simulink model "ChiefMaster_TTC580"  (R2022b)
settings: Solver=FixedStepAuto  StartTime=0.0  StopTime=10  FixedStep=0.01  RelTol=1e-3
values from neighbouring files (symbols this model uses):
  BattBox1_No = single(1)    [Parameters.m]
  BattBox2_No = single(2)    [Parameters.m]
  BattBox3_No = single(3)    [Parameters.m]
  CurrentLB = single(-3)    [Parameters.m]
  CurrentReductionConstant_Lvl0 = single(0.03)    [Parameters.m]
  CurrentReductionConstant_Lvl1 = single(0.05)    [Parameters.m]
  CurrentReductionConstant_Lvl2 = single(0.07)    [Parameters.m]
  CurrentReductionConstant_Lvl3 = single(0.1)    [Parameters.m]
  CurrentUB = single(3)    [Parameters.m]
  DCHV_Minus_In_Delay_ms = single(500)    [Parameters.m]
  FL_sHVC_CellBalanceVoltage_mV = single(3500)    [Parameters.m]
  FL_sInrushCurrent_dividebyzero = single(0.00001)    [Parameters.m]
  FL_u8HMI_BuzzerTimer = uint8(3)    [Parameters.m]
  IP_boActValue = true    [Parameters.m]
  IP_boDeactValue = false    [Parameters.m]
  IP_boInitValue = false    [Parameters.m]
  IP_s_LB = 18000    [Parameters.m]
  IP_s_UB = 22000    [Parameters.m]
  IP_sBatt1_ChargeCurrentMax_Factor = single(0.1)    [Parameters.m]
  IP_sBatt1_ChargeCurrentMax_LB = single(0)    [Parameters.m]
  IP_sBatt1_ChargeCurrentMax_Offset = single(0)    [Parameters.m]
  IP_sBatt1_ChargeCurrentMax_UB = single(6553.5)    [Parameters.m]
  IP_sBatt1_Current_Factor = single(0.1)    [Parameters.m]
  IP_sBatt1_Current_LB = single(-3276.8)    [Parameters.m]
  IP_sBatt1_Current_Offset = single(0)    [Parameters.m]
  IP_sBatt1_Current_UB = single(3276.8)    [Parameters.m]
  IP_sBatt1_DisChargeCurrentMax_Factor = single(0.1)    [Parameters.m]
  IP_sBatt1_DisChargeCurrentMax_LB = single(0)    [Parameters.m]
  IP_sBatt1_DisChargeCurrentMax_Offset = single(0)    [Parameters.m]
  IP_sBatt1_DisChargeCurrentMax_UB = single(6553.5)    [Parameters.m]
  IP_sBatt1_InsulationResistance_Factor = single(5)    [Parameters.m]
  IP_sBatt1_InsulationResistance_LB = single(0)    [Parameters.m]
  IP_sBatt1_InsulationResistance_Offset = single(0)    [Parameters.m]
  IP_sBatt1_InsulationResistance_UB = single(0)    [Parameters.m]
  IP_sBatt1_LiBa_IntResist_mOhm = single(25)    [Parameters.m]
  IP_sBatt1_SOC_Factor = single(1)    [Parameters.m]
  IP_sBatt1_SOC_LB = single(0)    [Parameters.m]
  IP_sBatt1_SOC_Offset = single(0)    [Parameters.m]
  IP_sBatt1_SOC_UB = single(100)    [Parameters.m]
  IP_sBatt1_SOH_Factor = single(1)    [Parameters.m]
  IP_sBatt1_SOH_LB = single(0)    [Parameters.m]
  IP_sBatt1_SOH_Offset = single(0)    [Parameters.m]
  IP_sBatt1_SOH_UB = single(100)    [Parameters.m]
  IP_sBatt1_Ubatt_Factor = single(0.1)    [Parameters.m]
  IP_sBatt1_Ubatt_LB = single(0)    [Parameters.m]
  IP_sBatt1_Ubatt_Offset = single(0)    [Parameters.m]
  IP_sBatt1_Ubatt_UB = single(6553.5)    [Parameters.m]
  IP_sBatt1_UserRi_Factor = single(1)    [Parameters.m]
  IP_sBatt1_UserRi_LB = single(0)    [Parameters.m]
  IP_sBatt1_UserRi_Offset = single(0)    [Parameters.m]
  IP_sBatt1_UserRi_UB = single(255)    [Parameters.m]
  IP_sBatt1_VoltageAtSensor_Factor = single(0.02)    [Parameters.m]
  IP_sBatt1_VoltageAtSensor_LB = single(0)    [Parameters.m]
  IP_sBatt1_VoltageAtSensor_Offset = single(0)    [Parameters.m]
  IP_sBatt1_VoltageAtSensor_UB = single(1310.7)    [Parameters.m]
  IP_sBatt2_LiBa_IntResist_mOhm = single(25)    [Parameters.m]
  IP_sBatt3_LiBa_IntResist_mOhm = single(25)    [Parameters.m]
  IP_sEM_LB = 2000    [Parameters.m]
  IP_sEM_UB = 8000    [Parameters.m]
  IP_sFB_LB = 5000    [Parameters.m]
  IP_sFB_UB = 10000    [Parameters.m]
  IP_sHVIL_LB = 12000    [Parameters.m]
  IP_sHVIL_UB = 15000    [Parameters.m]
  IP_sLoad_Voltage_Factor = single(1)    [Parameters.m]
  IP_sLoad_Voltage_LB = single(0)    [Parameters.m]
  IP_sLoad_Voltage_Offset = single(0)    [Parameters.m]
  IP_sLoad_Voltage_UB = single(65535)    [Parameters.m]
  IP_u8HVIL_Delay_ms = uint8(100)    [Parameters.m]
  IP_u8HW_IN_delay_ms = uint8(100)    [Parameters.m]
  IT_sInsulationSafeValue_kOhm = single(650)    [Parameters.m]
  IT_u8IMD_DelayTime_s = uint8(20)    [Parameters.m]
  MainHV_Minus_In_Delay = single(5)    [Parameters.m]
  MainHV_StatusDelay = single(5)    [Parameters.m]
  NotAvailable_uint16 = single(65535)    [Parameters.m]
  NotAvailable_uint8 = uint8(255)    [Parameters.m]
  OP_boHVIL_Supply = boolean(1)    [Parameters.m]
  SafeCurrentToCloseHV_A = single(5)    [Parameters.m]
  SafeVoltageToCloseHV_V = single(0.5)    [Parameters.m]
  UnexpectedBattChargingFcn_Available = boolean(1)    [Parameters.m]
  Voltage_NA_UB = uint16(65535)    [Parameters.m]
  VoltageSensorAvailableBB1 = boolean(0)    [Parameters.m]
  VoltageSensorAvailableBB2 = boolean(0)    [Parameters.m]
  VoltageSensorAvailableBB3 = boolean(0)    [Parameters.m]
libraries: simulink x184, Library_DataProcessing_v1_1 x167, Library_DataProcessing_v1 x142, libCM x28
(part 4 of 19)

== system ChiefMaster_TTC580/ChiefMaster/Input Translation/HW Inputs ==
  IP_Databus : Inport
  Bus Creator : BusCreator  Inputs=15
  Bus Selector : BusSelector  OutputSignals=IP_HW_Input_DataBus.IP_boHW_KL15,IP_HW_Input_DataBus.IP_boHW_HVIL_BDU,IP_HW_Input_DataBus.IP_boHW_HVIL_Components,IP_HW_Input_DataBus.IP_boHW_HVIL_Battery,IP_HW_Input_DataBus.IP_boHW_HVIL_Overrule,IP_HW_Input_DataBus.IP_boHW_MainHV_Plus_FB,IP_HW_Input_DataBus.IP_boHW_MainHV_Minus_FB,IP_HW_Input_DataBus.IP_boHW_EmergencyButton_NC,IP_HW_Input_DataBus.IP_boHW_EmergencyButton_NO,IP_HW_Input_DataBus.IP_boHW_ResetButton_LED_NO,IP_HW_Input_DataBus.IP_boHW_Proximity_BB1,IP_HW_Input_DataBus.IP_boHW_Proximity_BB2,IP_HW_Input_DataBus.IP_boHW_Proximity_BB3,IP_HW_Input_DataBus.IP_boHW_DCHV_Plus_FB,IP_HW_Input_DataBus.IP_boHW_DCHV_Minus_FB
  Signal Copy{,1..14} (15 alike) : SignalConversion  OverrideOpt=off
  IT_HW_Input_Databus : Outport
  wires:
  Signal Copy/1 -> Bus Creator/1  "IT_boHW_KL15"
  Signal Copy11/1 -> Bus Creator/13  "IT_boHW_Proximity_BB3"
  Bus Selector/8 -> Signal Copy6/1  "<IP_boHW_EmergencyButton_NC>"
  Bus Selector/4 -> Signal Copy3/1  "<IP_boHW_HVIL_Battery>"
  Signal Copy3/1 -> Bus Creator/4  "IT_boHW_HVIL_Battery"
  Bus Selector/10 -> Signal Copy8/1  "<IP_boHW_ResetButton_LED_NO>"
  Signal Copy9/1 -> Bus Creator/11  "IT_boHW_Proximity_BB1"
  Signal Copy1/1 -> Bus Creator/2  "IT_boHW_HVIL_BDU"
  Signal Copy4/1 -> Bus Creator/6  "IT_boHW_MainHV_Plus_FB"
  Signal Copy2/1 -> Bus Creator/3  "IT_boHW_HVIL_Components"
  Bus Selector/15 -> Signal Copy13/1  "<IP_boHW_DCHV_Minus_FB>"
  Signal Copy6/1 -> Bus Creator/8  "IT_sHW_EmergencyButton_NC"
  Bus Selector/6 -> Signal Copy4/1  "<IP_boHW_MainHV_Plus_FB>"
  Bus Selector/7 -> Signal Copy5/1  "<IP_boHW_MainHV_Minus_FB>"
  Bus Selector/12 -> Signal Copy10/1  "<IP_boHW_Proximity_BB2>"
  Bus Selector/3 -> Signal Copy2/1  "<IP_boHW_HVIL_Components>"
  Signal Copy12/1 -> Bus Creator/14  "IT_boHW_DCHV_Plus_FB"
  Signal Copy5/1 -> Bus Creator/7  "IT_boHW_MainHV_Minus_FB"
  Signal Copy13/1 -> Bus Creator/15  "IT_boHW_DCHV_Minus_FB"
  Bus Selector/9 -> Signal Copy7/1  "<IP_boHW_EmergencyButton_NO>"
  Bus Selector/11 -> Signal Copy9/1  "<IP_boHW_Proximity_BB1>"
  Bus Selector/14 -> Signal Copy12/1  "<IP_boHW_DCHV_Plus_FB>"
  Bus Selector/13 -> Signal Copy11/1  "<IP_boHW_Proximity_BB3>"
  Signal Copy10/1 -> Bus Creator/12  "IT_boHW_Proximity_BB2"
  Bus Selector/1 -> Signal Copy/1  "<IP_boHW_KL15>"
  Signal Copy7/1 -> Bus Creator/9  "IT_boHW_EmergencyButton_NO"
  Bus Selector/2 -> Signal Copy1/1  "<IP_boHW_HVIL_BDU>"
  Signal Copy8/1 -> Bus Creator/10  "IT_boHW_ResetButton_LED_NO"
  IP_Databus/1 -> Bus Selector/1
  Bus Creator/1 -> IT_HW_Input_Databus/1  "IT_HW_Input_Databus"
  Bus Selector/5 -> Signal Copy14/1  "<IP_boHW_HVIL_Overrule>"
  Signal Copy14/1 -> Bus Creator/5  "IT_boHW_HVIL_Overrule"

== system ChiefMaster_TTC580/ChiefMaster/Input Translation/UDC ==
  IP_Databus : Inport
  Bus Creator : BusCreator  Inputs=7
  Bus Selector : BusSelector  OutputSignals=UDC_Databus.IP_UDC_Status_Databus.IP_boSafeToShutdown,UDC_Databus.IP_UDC_Status_Databus.IP_boKL15_D,UDC_Databus.IP_UDC_Status_Databus.IP_boKL15_C,UDC_Databus.IP_UDC_Status_Databus.IP_boEVDisconnectingDevice,UDC_Databus.IP_UDC_Status_Databus.IP_boEV_IsolationMeasurementRequest,UDC_Databus.IP_UDC_Status_Databus.IP_boChargeStop_Button,UDC_Databus.IP_sLoadVoltage_Databus
  Bus Selector1 : BusSelector  OutputSignals=sData
  Signal Copy{,1..6} (7 alike) : SignalConversion  OverrideOpt=off
  IT_UDC_Databus : Outport
  wires:
  Bus Selector/1 -> Signal Copy/1  "<IP_boSafeToShutdown>"
  Signal Copy/1 -> Bus Creator/1  "IT_boUDC_SafeToShutdown"
  Bus Selector/3 -> Signal Copy2/1  "<IP_boKL15_C>"
  Signal Copy1/1 -> Bus Creator/2  "IT_boUDC_KL15_D"
  Bus Selector/2 -> Signal Copy1/1  "<IP_boKL15_D>"
  IP_Databus/1 -> Bus Selector/1
  Bus Selector1/1 -> Signal Copy3/1  "<sData>"
  Bus Selector/7 -> Bus Selector1/1  "<IP_sLoadVoltage_Databus>"
  Signal Copy2/1 -> Bus Creator/3  "IT_boUDC_KL15_C"
  Signal Copy3/1 -> Bus Creator/7  "IT_sUDC_LoadVoltage_V"
  Bus Creator/1 -> IT_UDC_Databus/1  "IT_UDC_Databus"
  Bus Selector/4 -> Signal Copy4/1  "<IP_boEVDisconnectingDevice>"
  Signal Copy4/1 -> Bus Creator/4  "IT_boUDC_EVDisconnectingDevice"
  Bus Selector/5 -> Signal Copy5/1  "<IP_boEV_IsolationMeasurementRequest>"
  Signal Copy5/1 -> Bus Creator/5  "IT_boUDC_EV_IsolationMeasurementRequest"
  Bus Selector/6 -> Signal Copy6/1  "<IP_boChargeStop_Button>"
  Signal Copy6/1 -> Bus Creator/6  "IT_boChargeStop_Button"

== system ChiefMaster_TTC580/ChiefMaster/Output Processing/CM_OBD ==
  OT_Databus : Inport
  CM_BDU_Msg5_6 : Subsystem
  CM_Battery1_Msg7 : Subsystem
  CM_Battery1_Msg8 : Subsystem
  CM_Battery1_Msg9 : Subsystem
  CM_Battery2_Msg10 : Subsystem
  CM_Battery2_Msg11 : Subsystem
  CM_Battery2_Msg12 : Subsystem
  CM_Battery3_Msg13 : Subsystem
  CM_Battery3_Msg14 : Subsystem
  CM_Battery3_Msg15 : Subsystem
  CM_IP_Msg1 : Subsystem
  CM_OP_Msg2 : Subsystem
  CM_SystemStatus1_Msg3 : Subsystem
  CM_SystemStatus2_Msg4 : Subsystem
  OP_ChiefMaster_IP_Msg1 : Outport
  OP_ChiefMaster_OP_Msg2 : Outport  Port=2
  OP_ChiefMaster_SS1_Msg3 : Outport  Port=3
  OP_ChiefMaster_SS2_Msg4 : Outport  Port=4
  OP_ChiefMaster_Calc_Msg5 : Outport  Port=5
  OP_ChiefMaster_BDU_Msg6 : Outport  Port=6
  OP_ChiefMaster_Battery1_Msg7 : Outport  Port=7
  OP_ChiefMaster_Battery1_Msg8 : Outport  Port=8
  OP_ChiefMaster_Battery1_Msg9 : Outport  Port=9
  OP_ChiefMaster_Battery2_Msg10 : Outport  Port=10
  OP_ChiefMaster_Battery2_Msg11 : Outport  Port=11
  OP_ChiefMaster_Battery2_Msg12 : Outport  Port=12
  OP_ChiefMaster_Battery3_Msg13 : Outport  Port=13
  OP_ChiefMaster_Battery3_Msg14 : Outport  Port=14
  OP_ChiefMaster_Battery3_Msg15 : Outport  Port=15
  wires:
  CM_SystemStatus1_Msg3/1(OP_ChiefMaster_SS_Msg3) -> OP_ChiefMaster_SS1_Msg3/1
  CM_SystemStatus2_Msg4/1(OP_ChiefMaster_SS2_Msg4) -> OP_ChiefMaster_SS2_Msg4/1
  CM_IP_Msg1/1(OP_ChiefMaster_IP_Msg1) -> OP_ChiefMaster_IP_Msg1/1
  CM_OP_Msg2/1(OP_ChiefMaster_OP_Msg2) -> OP_ChiefMaster_OP_Msg2/1
  CM_BDU_Msg5_6/1("Chief_Master_Calc_Msg5 ") -> OP_ChiefMaster_Calc_Msg5/1
  CM_BDU_Msg5_6/2(Chief_Master_BDU_Msg6) -> OP_ChiefMaster_BDU_Msg6/1
  CM_Battery1_Msg7/1(OP_ChiefMaster_Battery1_Msg7) -> OP_ChiefMaster_Battery1_Msg7/1
  CM_Battery1_Msg8/1(OP_ChiefMaster_Battery1_Msg8) -> OP_ChiefMaster_Battery1_Msg8/1
  CM_Battery2_Msg11/1(OP_ChiefMaster_Battery2_Msg10) -> OP_ChiefMaster_Battery2_Msg11/1
  CM_Battery2_Msg10/1(OP_ChiefMaster_Battery2_Msg9) -> OP_ChiefMaster_Battery2_Msg10/1
  OT_Databus/1 -> CM_IP_Msg1/1(OT_Databus), CM_OP_Msg2/1(OT_Databus), CM_SystemStatus1_Msg3/1(OT_Databus), CM_SystemStatus2_Msg4/1(OT_Databus), CM_BDU_Msg5_6/1(OT_Databus), CM_Battery1_Msg7/1(OT_Databus), CM_Battery3_Msg15/1(OT_Databus), CM_Battery3_Msg14/1(OT_Databus), CM_Battery3_Msg13/1(OT_Databus), CM_Battery2_Msg12/1(OT_Databus), CM_Battery2_Msg11/1(OT_Databus), CM_Battery2_Msg10/1(OT_Databus), CM_Battery1_Msg9/1(OT_Databus), CM_Battery1_Msg8/1(OT_Databus)
  CM_Battery3_Msg13/1(OP_ChiefMaster_Battery3_Msg11) -> OP_ChiefMaster_Battery3_Msg13/1
  CM_Battery3_Msg14/1(OP_ChiefMaster_Battery3_Msg12) -> OP_ChiefMaster_Battery3_Msg14/1
  CM_Battery1_Msg9/1(OP_ChiefMaster_Battery1_Msg8) -> OP_ChiefMaster_Battery1_Msg9/1
  CM_Battery2_Msg12/1(OP_ChiefMaster_Battery1_Msg8) -> OP_ChiefMaster_Battery2_Msg12/1
  CM_Battery3_Msg15/1(OP_ChiefMaster_Battery1_Msg8) -> OP_ChiefMaster_Battery3_Msg15/1

== system ChiefMaster_TTC580/ChiefMaster/Output Processing/OP_Actia ==
  OT_Databus : Inport
  Bus Selector1 : BusSelector  OutputSignals=OT_BatteryBox_HVControl_Databus.OT_boREQ_HV_ON_BB1,OT_IMD_Databus.OT_boREQ_IMD_ON_BB1
  Bus Selector2 : BusSelector  OutputSignals=OT_BatteryBox_HVControl_Databus.OT_boREQ_HV_ON_BB2,OT_IMD_Databus.OT_boREQ_IMD_ON_BB2
  Bus Selector3 : BusSelector  OutputSignals=OT_BatteryBox_HVControl_Databus.OT_boREQ_HV_ON_BB3,OT_IMD_Databus.OT_boREQ_IMD_ON_BB3
  Subsystem2 : Subsystem
  Subsystem3 : Subsystem
  Subsystem4 : Subsystem
  OP_Actia_Control_Batt1 : Outport
  OP_Actia_Control_Batt2 : Outport  Port=2
  OP_Actia_Control_Batt3 : Outport  Port=3
  wires:
  Bus Selector2/1 -> Subsystem3/1(<FL_boREQ_HV_ON_BB2>)  "<OT_boREQ_HV_ON_BB2>"
  Bus Selector3/1 -> Subsystem4/1(<FL_boREQ_HV_ON_BB3>)  "<OT_boREQ_HV_ON_BB3>"
  Bus Selector1/1 -> Subsystem2/1(<FL_boREQ_HV_ON_BB1>)  "<OT_boREQ_HV_ON_BB1>"
  Bus Selector2/2 -> Subsystem3/2(<FL_boREQ_IMD_ON_BB2>)  "<OT_boREQ_IMD_ON_BB2>"
  Bus Selector1/2 -> Subsystem2/2(<FL_boREQ_IMD_ON_BB1>)  "<OT_boREQ_IMD_ON_BB1>"
  Bus Selector3/2 -> Subsystem4/2(<FL_boREQ_IMD_ON_BB3>)  "<OT_boREQ_IMD_ON_BB3>"
  OT_Databus/1 -> Bus Selector1/1, Bus Selector3/1, Bus Selector2/1
  Subsystem2/1(OP_Actia_Control_Batt1) -> OP_Actia_Control_Batt1/1
  Subsystem3/1(OP_Actia_Control_Batt2) -> OP_Actia_Control_Batt2/1
  Subsystem4/1(OP_Actia_Control_Batt3) -> OP_Actia_Control_Batt3/1

== system ChiefMaster_TTC580/ChiefMaster/Output Processing/OP_HW ==
  OT_Databus : Inport
  Bus Selector : BusSelector  OutputSignals=OT_KL15_Databus.OT_boKL15_BB1,OT_KL15_Databus.OT_boKL15_BB2,OT_KL15_Databus.OT_boKL15_BB3,OT_BDUControl_Databus.OT_boREQ_MainHV_ON_MINUS,OT_BDUControl_Databus.OT_boREQ_MainHV_ON_PLUS,OT_BDUControl_Databus.OT_boREQ_MainHV_ON_Precharge,OT_BDUControl_Databus.OT_boREQ_DC_ON_MINUS,OT_BDUControl_Databus.OT_boREQ_DC_ON_Plus,OT_IMD_Databus.OT_boREQ_IMD_ON_BB1,OT_IMD_Databus.OT_boREQ_IMD_ON_BB2,OT_IMD_Databus.OT_boREQ_IMD_ON_BB3,OT_SystemStatus_Databus.OT_boSS_CabinAlarm,OT_SystemStatus_Databus.OT_boSS_EMSRET_POWER,OT_SystemStatus_Databus.OT_boSS_Resetbutton_LED
  Constant : Constant  Value=OP_boHVIL_Supply  OutDataTypeStr=boolean
  OT_boKL15_BB1 : Outport
  OT_boKL15_BB2 : Outport  Port=2
  OT_boKL15_BB3 : Outport  Port=3
  OT_boREQ_MainHV_ON_MINUS : Outport  Port=4
  OT_boREQ_MainHV_ON_PLUS : Outport  Port=5
  OT_boREQ_MainHV_ON_Precharge : Outport  Port=6
  OT_boREQ_DC_ON_MINUS : Outport  Port=7
  OT_boREQ_DC_ON_PLUS : Outport  Port=8
  OT_boKL15_IMD_BB1 : Outport  Port=9  OutDataTypeStr=boolean
  OT_boKL15_IMD_BB2 : Outport  Port=10  OutDataTypeStr=boolean
  OT_boKL15_IMD_BB3 : Outport  Port=11  OutDataTypeStr=boolean
  OT_CabinAlarm : Outport  Port=12
  OT_boEMSRET_BDU1 : Outport  Port=13  OutDataTypeStr=boolean
  OT_boEMSRET_BDU2 : Outport  Port=14  OutDataTypeStr=boolean
  OT_boEMSRET_BB1_1 : Outport  Port=15  OutDataTypeStr=boolean
  OT_boEMSRET_BB1_2 : Outport  Port=16  OutDataTypeStr=boolean
  OT_boEMSRET_BB2_1 : Outport  Port=17  OutDataTypeStr=boolean
  OT_boEMSRET_BB2_2 : Outport  Port=18  OutDataTypeStr=boolean
  OT_boEMSRET_BB3_1 : Outport  Port=19  OutDataTypeStr=boolean
  OT_boEMSRET_BB3_2 : Outport  Port=20  OutDataTypeStr=boolean
  OT_boHVIL_Supply : Outport  Port=21  OutDataTypeStr=boolean
  OT_boResetButton_LED : Outport  Port=22  OutDataTypeStr=boolean
  wires:
  Bus Selector/3 -> OT_boKL15_BB3/1  "<OT_boKL15_BB3>"
  OT_Databus/1 -> Bus Selector/1
  Bus Selector/2 -> OT_boKL15_BB2/1  "<OT_boKL15_BB2>"
  Bus Selector/1 -> OT_boKL15_BB1/1  "<OT_boKL15_BB1>"
  Bus Selector/5 -> OT_boREQ_MainHV_ON_PLUS/1  "<OT_boREQ_MainHV_ON_PLUS>"
  Bus Selector/4 -> OT_boREQ_MainHV_ON_MINUS/1  "<OT_boREQ_MainHV_ON_MINUS>"
  Bus Selector/6 -> OT_boREQ_MainHV_ON_Precharge/1  "<OT_boREQ_MainHV_ON_Precharge>"
  Bus Selector/7 -> OT_boREQ_DC_ON_MINUS/1  "<OT_boREQ_DC_ON_MINUS>"
  Bus Selector/8 -> OT_boREQ_DC_ON_PLUS/1  "<OT_boREQ_DC_ON_Plus>"
  Bus Selector/9 -> OT_boKL15_IMD_BB1/1  "<OT_boREQ_IMD_ON_BB1>"
  Bus Selector/10 -> OT_boKL15_IMD_BB2/1  "<OT_boREQ_IMD_ON_BB2>"
  Bus Selector/11 -> OT_boKL15_IMD_BB3/1  "<OT_boREQ_IMD_ON_BB3>"
  Bus Selector/12 -> OT_CabinAlarm/1  "<OT_boSS_CabinAlarm>"
  Bus Selector/13 -> OT_boEMSRET_BB2_1/1, OT_boEMSRET_BB3_1/1, OT_boEMSRET_BB3_2/1, OT_boEMSRET_BB2_2/1, OT_boEMSRET_BB1_2/1, OT_boEMSRET_BB1_1/1, OT_boEMSRET_BDU2/1, OT_boEMSRET_BDU1/1  "<OT_boSS_EMSRET_POWER>"
  Constant/1 -> OT_boHVIL_Supply/1
  Bus Selector/14 -> OT_boResetButton_LED/1  "<OT_boSS_Resetbutton_LED>"

== system ChiefMaster_TTC580/ChiefMaster/Output Processing/OP_LiBa ==
  OT_Databus : Inport
  UDC_BMS_OperationRequest1 : Subsystem
  UDC_BMS_OperationRequest2 : Subsystem
  UDC_BMS_OperationRequest3 : Subsystem
  OP_LiBa_Control_Batt1 : Outport
  OP_LiBa_Control_Batt2 : Outport  Port=2
  OP_LiBa_Control_Batt3 : Outport  Port=3
  wires:
  UDC_BMS_OperationRequest1/1(OP_UDC_BMS_OperationRequest) -> OP_LiBa_Control_Batt1/1
  OT_Databus/1 -> UDC_BMS_OperationRequest3/1(OT_Databus), UDC_BMS_OperationRequest2/1(OT_Databus), UDC_BMS_OperationRequest1/1(OT_Databus)
  UDC_BMS_OperationRequest2/1(OP_UDC_BMS_OperationRequest) -> OP_LiBa_Control_Batt2/1
  UDC_BMS_OperationRequest3/1(OP_UDC_BMS_OperationRequest) -> OP_LiBa_Control_Batt3/1

== system ChiefMaster_TTC580/ChiefMaster/Output Translation/BDUControl ==
  FL_Databus : Inport
  Bus Creator1 : BusCreator  Inputs=14
  Bus Selector1 : BusSelector  OutputSignals=FL_BDUControl_Databus.FL_boREQ_MainHV_ON_MINUS,FL_BDUControl_Databus.FL_boREQ_MainHV_ON_Precharge,FL_BDUControl_Databus.FL_boREQ_MainHV_ON_PLUS,FL_BDUControl_Databus.FL_u8MainHV_Minus_Status,FL_BDUControl_Databus.FL_u8MainHV_Plus_Status,FL_BDUControl_Databus.FL_boMainHV_Minus_Welded,FL_BDUControl_Databus.FL_boMainHV_Plus_Welded,FL_BDUControl_Databus.FL_u8Precharge_Status,FL_BDUControl_Databus.FL_boMainHV_WeldingCheckActive,FL_BDUControl_Databus.FL_u8WeldingDetection_Status,FL_BDUControl_Databus.FL_boREQ_DC_ON_MINUS,FL_BDUControl_Databus.FL_boREQ_DC_ON_Plus,FL_BDUControl_Databus.FL_u8DCHV_Minus_Status,FL_BDUControl_Databus.FL_u8DCHV_Plus_Status
  Signal Copy{1..14} (14 alike) : SignalConversion  OverrideOpt=off
  OT_BDUControl_Databus : Outport
  wires:
  Signal Copy10/1 -> Bus Creator1/10  "OT_u8WeldingDetection_Status"
  Signal Copy8/1 -> Bus Creator1/8  "OT_u8Precharge_Status"
  Signal Copy6/1 -> Bus Creator1/6  "OT_boMainHV_Minus_Welded"
  Signal Copy5/1 -> Bus Creator1/5  "OT_u8MainHV_Plus_Status"
  Bus Selector1/4 -> Signal Copy4/1  "<FL_u8MainHV_Minus_Status>"
  Signal Copy2/1 -> Bus Creator1/2  "OT_boREQ_MainHV_ON_Precharge"
  Bus Selector1/8 -> Signal Copy8/1  "<FL_u8Precharge_Status>"
  Bus Selector1/6 -> Signal Copy6/1  "<FL_boMainHV_Minus_Welded>"
  Signal Copy1/1 -> Bus Creator1/1  "OT_boREQ_MainHV_ON_MINUS"
  Bus Selector1/2 -> Signal Copy2/1  "<FL_boREQ_MainHV_ON_Precharge>"
  Bus Selector1/5 -> Signal Copy5/1  "<FL_u8MainHV_Plus_Status>"
  Bus Selector1/1 -> Signal Copy1/1  "<FL_boREQ_MainHV_ON_MINUS>"
  Signal Copy4/1 -> Bus Creator1/4  "OT_u8MainHV_Minus_Status"
  Signal Copy3/1 -> Bus Creator1/3  "OT_boREQ_MainHV_ON_PLUS"
  Bus Selector1/10 -> Signal Copy10/1  "<FL_u8WeldingDetection_Status>"
  Bus Selector1/3 -> Signal Copy3/1  "<FL_boREQ_MainHV_ON_PLUS>"
  Signal Copy7/1 -> Bus Creator1/7  "OT_boMainHV_Plus_Welded"
  Bus Selector1/9 -> Signal Copy9/1  "<FL_boMainHV_WeldingCheckActive>"
  Signal Copy9/1 -> Bus Creator1/9  "OT_boMainHV_WeldingCheckActive"
  Bus Selector1/7 -> Signal Copy7/1  "<FL_boMainHV_Plus_Welded>"
  FL_Databus/1 -> Bus Selector1/1
  Bus Creator1/1 -> OT_BDUControl_Databus/1  "OT_BDUControl_Databus"
  Bus Selector1/11 -> Signal Copy11/1  "<FL_boREQ_DC_ON_MINUS>"
  Bus Selector1/12 -> Signal Copy12/1  "<FL_boREQ_DC_ON_Plus>"
  Signal Copy11/1 -> Bus Creator1/11  "OT_boREQ_DC_ON_MINUS"
  Signal Copy12/1 -> Bus Creator1/12  "OT_boREQ_DC_ON_Plus"
  Bus Selector1/13 -> Signal Copy13/1  "<FL_u8DCHV_Minus_Status>"
  Bus Selector1/14 -> Signal Copy14/1  "<FL_u8DCHV_Plus_Status>"
  Signal Copy13/1 -> Bus Creator1/13  "OT_u8DCHV_Minus_Status"
  Signal Copy14/1 -> Bus Creator1/14  "OT_u8DCHV_plus_Status"

== system ChiefMaster_TTC580/ChiefMaster/Output Translation/BatteryBox ==
  FL_Databus : Inport
  Bus Creator1 : BusCreator  Inputs=9
  Bus Selector1 : BusSelector  OutputSignals=FL_BatteryBox_HVControl_Databus.FL_u8ContactorState_BB1,FL_BatteryBox_HVControl_Databus.FL_u8ContactorState_BB2,FL_BatteryBox_HVControl_Databus.FL_u8ContactorState_BB3,FL_BatteryBox_HVControl_Databus.FL_boREQ_HV_ON_BB1,FL_BatteryBox_HVControl_Databus.FL_boREQ_HV_ON_BB2,FL_BatteryBox_HVControl_Databus.FL_boREQ_HV_ON_BB3,FL_BatteryBox_HVControl_Databus.FL_u8Contactor_FB_State_BB1,FL_BatteryBox_HVControl_Databus.FL_u8Contactor_FB_State_BB2,FL_BatteryBox_HVControl_Databus.FL_u8Contactor_FB_State_BB3
  Signal Copy{,1..8} (9 alike) : SignalConversion  OverrideOpt=off
  OT_BatteryBox_HVControl_Databus : Outport
  wires:
  Signal Copy6/1 -> Bus Creator1/7  "OT_u8Contactor_FB_State_BB1"
  Bus Selector1/1 -> Signal Copy/1  "<FL_u8ContactorState_BB1>"
  Bus Selector1/5 -> Signal Copy4/1  "<FL_boREQ_HV_ON_BB2>"
  Signal Copy4/1 -> Bus Creator1/5  "OT_boREQ_HV_ON_BB2"
  Bus Selector1/3 -> Signal Copy2/1  "<FL_u8ContactorState_BB3>"
  Bus Selector1/8 -> Signal Copy7/1  "<FL_u8Contactor_FB_State_BB2>"
  Signal Copy3/1 -> Bus Creator1/4  "OT_boREQ_HV_ON_BB1"
  Signal Copy7/1 -> Bus Creator1/8  "OT_u8Contactor_FB_State_BB2"
  Bus Selector1/4 -> Signal Copy3/1  "<FL_boREQ_HV_ON_BB1>"
  Signal Copy2/1 -> Bus Creator1/3  "OT_u8ContactorState_BB3"
  Signal Copy5/1 -> Bus Creator1/6  "OT_boREQ_HV_ON_BB3"
  Signal Copy1/1 -> Bus Creator1/2  "OT_u8ContactorState_BB2"
  Signal Copy/1 -> Bus Creator1/1  "OT_u8ContactorState_BB1"
  Bus Selector1/2 -> Signal Copy1/1  "<FL_u8ContactorState_BB2>"
  Bus Selector1/9 -> Signal Copy8/1  "<FL_u8Contactor_FB_State_BB3>"
  Bus Creator1/1 -> OT_BatteryBox_HVControl_Databus/1  "OT_BatteryBox_HVControl_Databus"
  Signal Copy8/1 -> Bus Creator1/9  "OT_u8Contactor_FB_State_BB3"
  Bus Selector1/7 -> Signal Copy6/1  "<FL_u8Contactor_FB_State_BB1>"
  Bus Selector1/6 -> Signal Copy5/1  "<FL_boREQ_HV_ON_BB3>"
  FL_Databus/1 -> Bus Selector1/1

== system ChiefMaster_TTC580/ChiefMaster/Output Translation/IMD ==
  FL_Databus : Inport
  Bus Creator1 : BusCreator  Inputs=6
  Bus Selector : BusSelector  OutputSignals=FL_IMD_Control_Databus.FL_boREQ_IMD_ON_BB1,FL_IMD_Control_Databus.FL_boREQ_IMD_ON_BB2,FL_IMD_Control_Databus.FL_boREQ_IMD_ON_BB3,FL_IMD_Control_Databus.FL_u8_IMD_State_BB1,FL_IMD_Control_Databus.FL_u8_IMD_State_BB2,FL_IMD_Control_Databus.FL_u8_IMD_State_BB3
  Signal Copy : SignalConversion  OverrideOpt=off
  Signal Copy1 : SignalConversion  OverrideOpt=off
  Signal Copy2 : SignalConversion  OverrideOpt=off
  Subsystem : Subsystem
  Subsystem1 : Subsystem
  Subsystem2 : Subsystem
  OT_IMD_Databus : Outport
  wires:
  Bus Selector/2 -> Subsystem1/1(<FL_boREQ_IMD_ON_BB2>)  "<FL_boREQ_IMD_ON_BB2>"
  Bus Creator1/1 -> OT_IMD_Databus/1  "OT_IMD_Databus"
  Bus Selector/1 -> Subsystem/1(<FL_boREQ_IMD_ON_BB1>)  "<FL_boREQ_IMD_ON_BB1>"
  Subsystem2/1(OT_boREQ_IMD_ON_BB3) -> Bus Creator1/3
  Subsystem1/1(OT_boREQ_IMD_ON_BB2) -> Bus Creator1/2
  Subsystem/1(OT_boREQ_IMD_ON_BB1) -> Bus Creator1/1
  Bus Selector/3 -> Subsystem2/1(<FL_boREQ_IMD_ON_BB3>)  "<FL_boREQ_IMD_ON_BB3>"
  FL_Databus/1 -> Bus Selector/1
  Bus Selector/4 -> Signal Copy/1  "<FL_u8_IMD_State_BB1>"
  Bus Selector/5 -> Signal Copy1/1  "<FL_u8_IMD_State_BB2>"
  Bus Selector/6 -> Signal Copy2/1  "<FL_u8_IMD_State_BB3>"
  Signal Copy/1 -> Bus Creator1/4  "OT_u8_IMD_State_BB1"
  Signal Copy1/1 -> Bus Creator1/5  "OT_u8_IMD_State_BB2"
  Signal Copy2/1 -> Bus Creator1/6  "OT_u8_IMD_State_BB3"

== system ChiefMaster_TTC580/ChiefMaster/Output Translation/KL15 ==
  FL_Databus : Inport
  Bus Creator : BusCreator  Inputs=3
  Bus Selector : BusSelector  OutputSignals=FL_KL15_Databus.FL_boKL15_BB1,FL_KL15_Databus.FL_boKL15_BB2,FL_KL15_Databus.FL_boKL15_BB3
  Signal Copy1 : SignalConversion  OverrideOpt=off
  Signal Copy2 : SignalConversion  OverrideOpt=off
  Signal Copy3 : SignalConversion  OverrideOpt=off
  OT_KL15_Databus : Outport
  wires:
  Bus Selector/1 -> Signal Copy1/1  "<FL_boKL15_BB1>"
  Bus Selector/3 -> Signal Copy3/1  "<FL_boKL15_BB3>"
  Bus Selector/2 -> Signal Copy2/1  "<FL_boKL15_BB2>"
  Signal Copy2/1 -> Bus Creator/2  "OT_boKL15_BB2"
  Signal Copy1/1 -> Bus Creator/1  "OT_boKL15_BB1"
  Signal Copy3/1 -> Bus Creator/3  "OT_boKL15_BB3"
  FL_Databus/1 -> Bus Selector/1
  Bus Creator/1 -> OT_KL15_Databus/1  "OT_KL15_Databus"

== system ChiefMaster_TTC580/ChiefMaster/Output Translation/SystemStatus ==
  FL_Databus : Inport
  Bus Creator : BusCreator  Inputs=21
  Bus Selector1 : BusSelector  OutputSignals=FL_SystemStatus_Databus.FL_u8SS_ChiefMaster_State,FL_SystemStatus_Databus.FL_boSS_System_Error,FL_SystemStatus_Databus.FL_u8SS_System_ErrorCode,FL_SystemStatus_Databus.FL_boSS_System_SD,FL_SystemStatus_Databus.FL_u8SS_System_SD_ErrorCode,FL_SystemStatus_Databus.FL_boSS_HVIL_NOK,FL_SystemStatus_Databus.FL_boSS_System_ESD,FL_SystemStatus_Databus.FL_u8SS_EmergencyStopState,FL_SystemStatus_Databus.FL_sSS_MaxChargeCurrent,FL_SystemStatus_Databus.FL_sSS_MaxDisChargeCurrent,FL_SystemStatus_Databus.FL_u8SS_SystemSOC,FL_SystemStatus_Databus.FL_sSS_System_Current,FL_SystemStatus_Databus.FL_sSS_SystemVoltage,FL_SystemStatus_Databus.FL_u8SS_NumberOfConnectedBatt,FL_SystemStatus_Databus.FL_boSS_BDU_Reset,FL_SystemStatus_Databus.FL_boSS_Batt_Warning,FL_SystemStatus_Databus.FL_boSS_Batt_Error,FL_SystemStatus_Databus.FL_boSS_Batt_SDError,FL_SystemStatus_Databus.FL_boSS_CabinAlarm,FL_SystemStatus_Databus.FL_boSS_EMSRET_POWER,FL_SystemStatus_Databus.FL_boSS_ResetButton_LED
  Signal Copy{,1..20} (21 alike) : SignalConversion  OverrideOpt=off
  OT_SystemStatus_Databus : Outport
  wires:
  Bus Selector1/17 -> Signal Copy16/1  "<FL_boSS_Batt_Error>"
  Bus Selector1/3 -> Signal Copy/1  "<FL_u8SS_System_ErrorCode>"
  Bus Selector1/1 -> Signal Copy1/1  "<FL_u8SS_ChiefMaster_State>"
  Bus Selector1/18 -> Signal Copy17/1  "<FL_boSS_Batt_SDError>"
  Bus Selector1/15 -> Signal Copy14/1  "<FL_boSS_BDU_Reset>"
  Bus Selector1/7 -> Signal Copy6/1  "<FL_boSS_System_ESD>"
  Bus Selector1/14 -> Signal Copy13/1  "<FL_u8SS_NumberOfConnectedBatt>"
  Bus Selector1/13 -> Signal Copy12/1  "<FL_sSS_SystemVoltage>"
  Bus Selector1/4 -> Signal Copy4/1  "<FL_boSS_System_SD>"
  Bus Selector1/16 -> Signal Copy15/1  "<FL_boSS_Batt_Warning>"
  Bus Selector1/5 -> Signal Copy5/1  "<FL_u8SS_System_SD_ErrorCode>"
  Bus Selector1/2 -> Signal Copy2/1  "<FL_boSS_System_Error>"
  Bus Selector1/8 -> Signal Copy7/1  "<FL_u8SS_EmergencyStopState>"
  Bus Selector1/9 -> Signal Copy8/1  "<FL_sSS_MaxChargeCurrent>"
  Bus Selector1/10 -> Signal Copy9/1  "<FL_sSS_MaxDisChargeCurrent>"
  Bus Selector1/11 -> Signal Copy10/1  "<FL_u8SS_SystemSOC>"
  Bus Selector1/12 -> Signal Copy11/1  "<FL_sSS_System_Current>"
  FL_Databus/1 -> Bus Selector1/1
  Signal Copy1/1 -> Bus Creator/1  "OT_u8SS_ChiefMaster_State"
  Signal Copy2/1 -> Bus Creator/2  "OT_boSS_System_Error"
  Signal Copy/1 -> Bus Creator/3  "OT_u8SS_System_ErrorCode"
  Signal Copy4/1 -> Bus Creator/4  "OT_boSS_System_SD"
  Signal Copy5/1 -> Bus Creator/5  "OT_u8SS_System_SD_ErrorCode"
  Signal Copy6/1 -> Bus Creator/7  "OT_boSS_System_ESD"
  Signal Copy7/1 -> Bus Creator/8  "OT_u8SS_EmergencyStopState"
  Signal Copy8/1 -> Bus Creator/9  "OT_sSS_MaxChargeCurrent"
  Signal Copy9/1 -> Bus Creator/10  "OT_sSS_MaxDisChargeCurrent"
  Signal Copy10/1 -> Bus Creator/11  "OT_u8SS_SystemSOC"
  Signal Copy11/1 -> Bus Creator/12  "OT_sSS_System_Current"
  Signal Copy12/1 -> Bus Creator/13  "OT_sSS_SystemVoltage"
  Signal Copy13/1 -> Bus Creator/14  "OT_u8SS_NumberOfConnectedBatt"
  Signal Copy14/1 -> Bus Creator/15  "OT_boSS_BDU_Reset"
  Signal Copy15/1 -> Bus Creator/16  "OT_boSS_Batt_Warning"
  Signal Copy16/1 -> Bus Creator/17  "OT_boSS_Batt_Error"
  Signal Copy17/1 -> Bus Creator/18  "OT_boSS_Batt_SDError"
  Bus Creator/1 -> OT_SystemStatus_Databus/1  "OT_SystemStatus_Databus"
  Bus Selector1/6 -> Signal Copy3/1  "<FL_boSS_HVIL_NOK>"
  Signal Copy3/1 -> Bus Creator/6  "OT_boSS_HVIL_NOK"
  Bus Selector1/19 -> Signal Copy18/1  "<FL_boSS_CabinAlarm>"
  Signal Copy18/1 -> Bus Creator/19  "OT_boSS_CabinAlarm"
  Bus Selector1/20 -> Signal Copy19/1  "<FL_boSS_EMSRET_POWER>"
  Signal Copy19/1 -> Bus Creator/20  "OT_boSS_EMSRET_POWER"
  Bus Selector1/21 -> Signal Copy20/1  "<FL_boSS_ResetButton_LED>"
  Signal Copy20/1 -> Bus Creator/21  "OT_boSS_Resetbutton_LED"

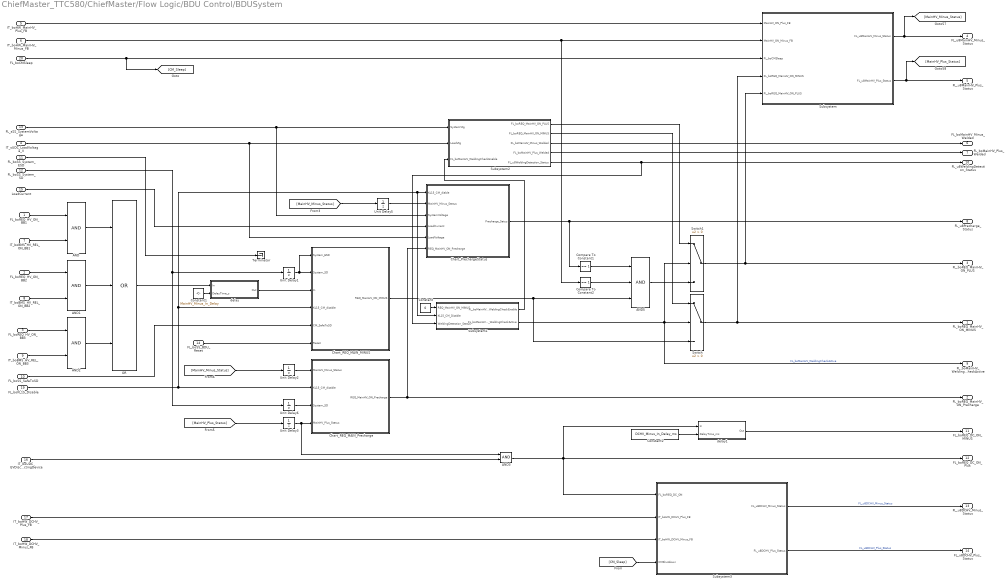
== system ChiefMaster_TTC580/ChiefMaster/Flow Logic/BDU Control/BDUSystem ==
  FL_boREQ_HV_ON_BB1 : Inport
  FL_boREQ_HV_ON_BB2 : Inport  Port=2
  FL_boREQ_HV_ON_BB3 : Inport  Port=3
  IT_sUDC_LoadVoltage_V : Inport  Port=4
  IT_boHW_MainHV_Plus_FB : Inport  Port=5
  IT_boHW_MainHV_Minus_FB : Inport  Port=6
  IT_boBMS_HV_REL_ON_BB1 : Inport  Port=7
  IT_boBMS_HV_REL_ON_BB2 : Inport  Port=8
  IT_boBMS_HV_REL_ON_BB3 : Inport  Port=9
  FL_boSS_SafeToSD : Inport  Port=10
  FL_boSS_System_ESD : Inport  Port=11
  FL_boSS_System_SD : Inport  Port=12
  FL_sSS_SystemVoltage : Inport  Port=13
  FL_boSS_BDU_Reset : Inport  Port=14
  LoadCurrent : Inport  Port=15
  IT_boUDC_EVDisconnectingDevice : Inport  Port=16
  IT_boHW_DCHV_Plus_FB : Inport  Port=17
  IT_boHW_DCHV_Minus_FB : Inport  Port=18
  FL_boKL15_Disable : Inport  Port=19
  FL_boCMSleep : Inport  Port=20
  AND{,1..3} (4 alike) : Logic  AllPortsSameDT=off  OutDataTypeStr=boolean
  AND5 : Logic  Inputs=3  AllPortsSameDT=off  OutDataTypeStr=boolean
  Chart_PrechargeStatus : Stateflow chart  TreatAsAtomicUnit=on
      settings: RTWSystemCode=Reusable function  RTWFcnNameOpts=Use subsystem name  RTWFileNameOpts=Use subsystem name  PortSchema="{\"entries\":[{\"content\":{\"sides\":[{\"content\":{\"connectorIds\":[\"In5\",\"In6\",\"In4\",\"In2\",\"In3\",\"In1\"]},\"type\":\"ConnectorPlacement.EquallySpacedRectSide\",\"uuid\":\"6cb37c1b-6d01-4332-a177-797190e5b6d6\"},{\"content\":{\"connectorIds\":[\"Out1\"],\"side\":\"RIGHT\"},\"type\":\"ConnectorPlacement.EquallySpacedRectSide\",\"uuid\":\"4e744c9a-40df-4e7e-bc86-0fe2b874664a\"},{\"content\":{\"connectorIds\":[],\"side\":\"TOP\"},\"type\":\"ConnectorPlacement.EquallySpacedRectSide\",\"uuid\":\"ec204ca1-0e33-4832-b6fe-b36fd4bcf128\"}]},\"type\":\"ConnectorPlacement.EquallySpacedConnector\",\"uuid\":\"41a36a0e-a0fa-4852-9cfa-238df43534ab\"}],\"packageUris\":[\"http://schema.mathworks.com/mf0/Connector/R2020b\"],\"version\":\"1.0\"}"
  Chart_REQ_MAIN_MINUS : Stateflow chart  TreatAsAtomicUnit=on
      settings: RTWSystemCode=Reusable function  RTWFcnNameOpts=Use subsystem name  RTWFileNameOpts=Use subsystem name  PortSchema="{\"entries\":[{\"content\":{\"sides\":[{\"content\":{\"connectorIds\":[\"In4\",\"In5\",\"In1\",\"In3\",\"In2\",\"In6\"]},\"type\":\"ConnectorPlacement.EquallySpacedRectSide\",\"uuid\":\"5f3eca62-e3d8-4efd-a1f1-61200c1e6bae\"},{\"content\":{\"connectorIds\":[\"Out1\"],\"side\":\"RIGHT\"},\"type\":\"ConnectorPlacement.EquallySpacedRectSide\",\"uuid\":\"169db87e-373b-4c5f-9f66-834028baf8aa\"},{\"content\":{\"connectorIds\":[],\"side\":\"TOP\"},\"type\":\"ConnectorPlacement.EquallySpacedRectSide\",\"uuid\":\"061e2ae4-d375-4149-b2d1-2bfb16532c6f\"}]},\"type\":\"ConnectorPlacement.EquallySpacedConnector\",\"uuid\":\"7b41504d-10e8-44e3-b1ad-70c8061d25ad\"}],\"packageUris\":[\"http://schema.mathworks.com/mf0/Connector/R2020b\"],\"version\":\"1.0\"}"
  Chart_REQ_MAIN_Precharge : Stateflow chart
      settings: RTWSystemCode=Reusable function  RTWFcnNameOpts=Use subsystem name  RTWFileNameOpts=Use subsystem name
  Compare To Constant1 : simulink/Logic and Bit Operations/Compare To Constant  relop===  const=1  OutDataTypeStr=boolean
  Compare To Constant2 : simulink/Logic and Bit Operations/Compare To Constant  relop===  const=1  OutDataTypeStr=boolean
  Constant : Constant  Value=0
  Constant1 : Constant  Value=MainHV_Minus_In_Delay
  Constant2 : Constant  Value=DCHV_Minus_In_Delay_ms
  OR : Logic  Operator=OR  Inputs=3  AllPortsSameDT=off  OutDataTypeStr=boolean
  Subsystem : Subsystem
  Subsystem1 : Subsystem
  Subsystem2 : Subsystem
  Subsystem3 : Subsystem
  Switch : Switch  Criteria=u2 > Threshold  SaturateOnIntegerOverflow=off  InputSameDT=off
  Switch1 : Switch  Criteria=u2 > Threshold  SaturateOnIntegerOverflow=off  InputSameDT=off
  Terminator : Terminator
  Unit Delay{1..3,5..6} (5 alike) : UnitDelay  SampleTime=-1  HasFrameUpgradeWarning=on
  delay : Stateflow chart  TreatAsAtomicUnit=on
  delay1 : Stateflow chart  TreatAsAtomicUnit=on
  FL_boREQ_MainHV_ON_MINUS : Outport
  FL_boREQ_MainHV_ON_Precharge : Outport  Port=2
  FL_boREQ_MainHV_ON_PLUS : Outport  Port=3
  FL_u8MainHV_Minus_Status : Outport  Port=4
  FL_u8MainHV_Plus_Status : Outport  Port=5
  FL_boMainHV_Minus_Welded : Outport  Port=6
  FL_boMainHV_Plus_Welded : Outport  Port=7
  FL_u8Precharge_Status : Outport  Port=8
  FL_boMainHV_WeldingCheckActive : Outport  Port=9
  FL_u8WeldingDetection_Status : Outport  Port=10
  FL_boREQ_DC_ON_MINUS : Outport  Port=11
  FL_boREQ_DC_ON_Plus : Outport  Port=12
  FL_u8DCHV_Minus_Status : Outport  Port=13
  FL_u8DCHV_Plus_Status : Outport  Port=14
  wires:
  FL_boREQ_HV_ON_BB2/1 -> AND1/1
  AND1/1 -> OR/2
  FL_boSS_System_SD/1 -> Unit Delay6/1, Unit Delay1/1
  Unit Delay3/1 -> AND3/1, Chart_REQ_MAIN_Precharge/4(MainHV_Plus_Status)
  [MainHV_Minus_Status] -> Unit Delay5/1
  FL_sSS_SystemVoltage/1 -> Chart_PrechargeStatus/4(SystemVoltage), Subsystem2/1(SystemVtg)
  FL_boSS_SafeToSD/1 -> Chart_REQ_MAIN_MINUS/2(CM_SafeToSD)
  IT_sUDC_LoadVoltage_V/1 -> Chart_PrechargeStatus/3(LoadVoltage), Subsystem2/2(LoadVtg)
  IT_boBMS_HV_REL_ON_BB3/1 -> AND2/2
  OR/1 -> delay/1(In)
  AND2/1 -> OR/3
  LoadCurrent/1 -> Chart_PrechargeStatus/2(LoadCurrent)
  AND/1 -> OR/1
  FL_boREQ_HV_ON_BB1/1 -> AND/1
  Subsystem2/4(FL_boMainHV_Plus_Welded) -> FL_boMainHV_Plus_Welded/1
  FL_boSS_System_ESD/1 -> Terminator/1
  FL_boSS_BDU_Reset/1 -> Chart_REQ_MAIN_MINUS/6(Reset)
  Constant/1 -> Subsystem1/1(REQ_MainHV_ON_MINUS)
  Subsystem/2(FL_u8MainHV_Plus_Status) -> [MainHV_Plus_Status], FL_u8MainHV_Plus_Status/1
  Chart_REQ_MAIN_Precharge/1(REQ_MainHV_ON_Precharge) -> Chart_PrechargeStatus/1(REQ_MainHV_ON_Precharge), FL_boREQ_MainHV_ON_Precharge/1
  IT_boBMS_HV_REL_ON_BB2/1 -> AND1/2
  Compare To Constant1/1 -> AND5/1
  Subsystem2/2(FL_boREQ_MainHV_ON_MINUS) -> Switch/1
  FL_boREQ_HV_ON_BB3/1 -> AND2/1
  AND5/1 -> Switch1/3
  IT_boHW_MainHV_Plus_FB/1 -> Subsystem/1(MainHV_ON_Plus_FB)
  Subsystem1/2(FL_boMainHV_WeldingCheckActive) -> Switch1/2, FL_boMainHV_WeldingCheckActive/1, Switch/2  "FL_boMainHV_WeldingCheckActive"
  IT_boBMS_HV_REL_ON_BB1/1 -> AND/2
  delay/1(Out) -> Chart_REQ_MAIN_MINUS/1(In)
  Chart_PrechargeStatus/1(Precharge_Satus) -> Compare To Constant1/1, FL_u8Precharge_Status/1
  [MainHV_Plus_Status] -> Unit Delay3/1
  Chart_REQ_MAIN_MINUS/1(REQ_MainHV_ON_MINUS) -> Switch/3, AND5/3
  Constant1/1 -> delay/2(DelayTime_s)
  FL_boKL15_Disable/1 -> Chart_REQ_MAIN_Precharge/2(KL15_CM_disable), Chart_REQ_MAIN_MINUS/3(KL15_CM_disable), Chart_PrechargeStatus/5(KL15_CM_diable), Subsystem1/2(KL15_CM_Disable)
  Switch/1 -> Subsystem/4(FL_boREQ_MainHV_ON_MINUS), FL_boREQ_MainHV_ON_MINUS/1
  Subsystem2/5(FL_u8WeldingDetection_Status) -> Subsystem1/3(WeldingDetection_Status), FL_u8WeldingDetection_Status/1
  Subsystem1/1(FL_boMainHV_WeldingCheckEnable) -> Subsystem2/3(FL_boMainHV_WeldingCheckEnable)
  Subsystem/1(FL_u8MainHV_Minus_Status) -> [MainHV_Minus_Status], FL_u8MainHV_Minus_Status/1
  Subsystem2/3(FL_boMainHV_Minus_Welded) -> FL_boMainHV_Minus_Welded/1
  IT_boHW_MainHV_Minus_FB/1 -> Compare To Constant2/1, Subsystem/2(MainHV_ON_Minus_FB)
  Subsystem2/1(FL_boREQ_MainHV_ON_PLUS) -> Switch1/1
  Unit Delay1/1 -> Chart_REQ_MAIN_MINUS/4(System_ESD), Chart_REQ_MAIN_MINUS/5(System_SD)
  Unit Delay6/1 -> Chart_REQ_MAIN_Precharge/3(System_SD)
  Compare To Constant2/1 -> AND5/2
  Unit Delay5/1 -> Chart_PrechargeStatus/6(MainHV_Minus_Status)
  Switch1/1 -> Subsystem/5(FL_boREQ_MainHV_ON_PLUS), FL_boREQ_MainHV_ON_PLUS/1
  [MainHV_Minus_Status] -> Unit Delay2/1
  Unit Delay2/1 -> Chart_REQ_MAIN_Precharge/1(MainHV_Minus_Status)
  FL_boCMSleep/1 -> [CM_Sleep], Subsystem/3(FL_boCMSleep)
  AND3/1 -> delay1/1(In), FL_boREQ_DC_ON_Plus/1, Subsystem3/1(FL_boREQ_DC_ON)
  IT_boHW_DCHV_Plus_FB/1 -> Subsystem3/2(IT_boHW_DCHV_Plus_FB)
  IT_boHW_DCHV_Minus_FB/1 -> Subsystem3/3(IT_boHW_DCHV_Minus_FB)
  IT_boUDC_EVDisconnectingDevice/1 -> AND3/2
  [CM_Sleep] -> Subsystem3/4(CMShutdown)
  Subsystem3/2(FL_u8DCHV_Plus_Status) -> FL_u8DCHV_Plus_Status/1  "FL_u8DCHV_Plus_Status"
  Subsystem3/1(FL_u8DCHV_Minus_Status) -> FL_u8DCHV_Minus_Status/1  "FL_u8DCHV_Minus_Status"
  delay1/1(Out) -> FL_boREQ_DC_ON_MINUS/1
  Constant2/1 -> delay1/2(DelayTime_ms)

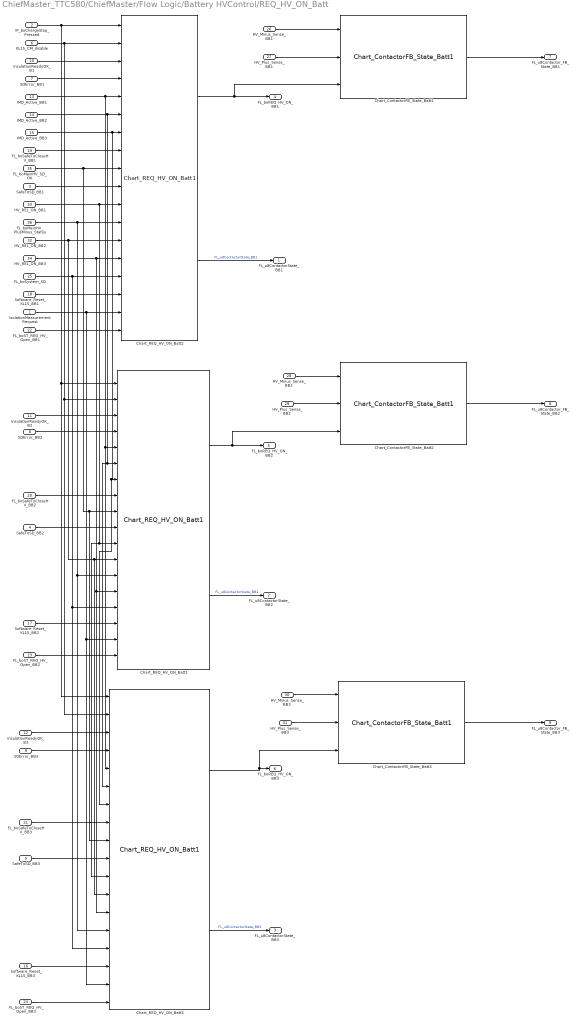
== system ChiefMaster_TTC580/ChiefMaster/Flow Logic/Battery HVControl/REQ_HV_ON_Batt ==
  IsolationMeasurementRequest : Inport
  IP_boChargeStop_Pressed : Inport  Port=2
  SafeToSD_BB1 : Inport  Port=3
  SafeToSD_BB2 : Inport  Port=4
  SafeToSD_BB3 : Inport  Port=5
  KL15_CM_disable : Inport  Port=6
  SDError_BB1 : Inport  Port=7
  SDError_BB2 : Inport  Port=8
  SDError_BB3 : Inport  Port=9
  InsulationReadyOK_B1 : Inport  Port=10
  InsulationReadyOK_B2 : Inport  Port=11
  InsulationReadyOK_B3 : Inport  Port=12
  IMD_Active_BB1 : Inport  Port=13
  IMD_Active_BB2 : Inport  Port=14
  IMD_Active_BB3 : Inport  Port=15
  Software_Reset_KL15_BB3 : Inport  Port=16
  Software_Reset_KL15_BB2 : Inport  Port=17
  Software_Reset_KL15_BB1 : Inport  Port=18
  FL_boSafeToCloseHV_BB1 : Inport  Port=19
  FL_boSafeToCloseHV_BB2 : Inport  Port=20
  FL_boSafeToCloseHV_BB3 : Inport  Port=21
  FL_boST_REQ_HV_Open_BB1 : Inport  Port=22
  FL_boST_REQ_HV_Open_BB2 : Inport  Port=23
  FL_boST_REQ_HV_Open_BB3 : Inport  Port=24
  FL_boSystem_SD : Inport  Port=25
  HV_Minus_Sense_BB1 : Inport  Port=26
  HV_Plus_Sense_BB1 : Inport  Port=27
  HV_Minus_Sense_BB2 : Inport  Port=28
  HV_Plus_Sense_BB2 : Inport  Port=29
  HV_Minus_Sense_BB3 : Inport  Port=30
  HV_Plus_Sense_BB3 : Inport  Port=31
  HV_REL_ON_BB2 : Inport  Port=32
  HV_REL_ON_BB1 : Inport  Port=33
  HV_REL_ON_BB3 : Inport  Port=34
  FL_boMainHV_SD_OK : Inport  Port=35
  FL_boMainHV_PlusMinus_Status : Inport  Port=36
  Chart_ContactorFB_State_Batt1 : libCM/Chart_ContactorFB_State_Batt1  SystemSampleTime=-1  VariantActivationTime=update diagram  Latency=0  AutoFrameSizeCalculation=off
  Chart_ContactorFB_State_Batt2 : libCM/Chart_ContactorFB_State_Batt1  SystemSampleTime=-1  VariantActivationTime=update diagram  Latency=0  AutoFrameSizeCalculation=off
  Chart_ContactorFB_State_Batt3 : libCM/Chart_ContactorFB_State_Batt1  SystemSampleTime=-1  VariantActivationTime=update diagram  Latency=0  AutoFrameSizeCalculation=off
  Chart_REQ_HV_ON_Batt1 : libCM/Chart_REQ_HV_ON_Batt1  SystemSampleTime=-1  VariantActivationTime=update diagram  Latency=0  AutoFrameSizeCalculation=off
      settings: PortSchema="{\"entries\":[{\"content\":{\"sides\":[{\"content\":{\"connectorIds\":[\"In1\",\"In8\",\"In2\",\"In3\",\"In4\",\"In5\",\"In6\",\"In9\",\"In10\",\"In11\",\"In15\",\"In16\",\"In12\",\"In13\",\"In14\",\"In7\",\"In17\",\"In18\"]},\"type\":\"ConnectorPlacement.EquallySpacedRectSide\",\"uuid\":\"2be98496-94d0-443a-935f-4b2e992aab8e\"},{\"content\":{\"connectorIds\":[\"Out1\",\"Out2\"],\"side\":\"RIGHT\"},\"type\":\"ConnectorPlacement.EquallySpacedRectSide\",\"uuid\":\"fda23760-2911-4bbb-ac8a-7a2dd70a4d72\"},{\"content\":{\"connectorIds\":[],\"side\":\"TOP\"},\"type\":\"ConnectorPlacement.EquallySpacedRectSide\",\"uuid\":\"77874347-bb9f-447e-8cfd-08f52997a658\"}]},\"type\":\"ConnectorPlacement.EquallySpacedConnector\",\"uuid\":\"fcafe625-79d7-4037-9431-d1cc167f79ab\"}],\"packageUris\":[\"http://schema.mathworks.com/mf0/Connector/R2020b\"],\"version\":\"1.0\"}"
  Chart_REQ_HV_ON_Batt2 : libCM/Chart_REQ_HV_ON_Batt1  SystemSampleTime=-1  VariantActivationTime=update diagram  Latency=0  AutoFrameSizeCalculation=off
      settings: PortSchema="{\"entries\":[{\"content\":{\"sides\":[{\"content\":{\"connectorIds\":[\"In1\",\"In8\",\"In2\",\"In3\",\"In4\",\"In5\",\"In6\",\"In9\",\"In10\",\"In11\",\"In15\",\"In16\",\"In12\",\"In13\",\"In14\",\"In7\",\"In17\",\"In18\"]},\"type\":\"ConnectorPlacement.EquallySpacedRectSide\",\"uuid\":\"2be98496-94d0-443a-935f-4b2e992aab8e\"},{\"content\":{\"connectorIds\":[\"Out1\",\"Out2\"],\"side\":\"RIGHT\"},\"type\":\"ConnectorPlacement.EquallySpacedRectSide\",\"uuid\":\"fda23760-2911-4bbb-ac8a-7a2dd70a4d72\"},{\"content\":{\"connectorIds\":[],\"side\":\"TOP\"},\"type\":\"ConnectorPlacement.EquallySpacedRectSide\",\"uuid\":\"77874347-bb9f-447e-8cfd-08f52997a658\"}]},\"type\":\"ConnectorPlacement.EquallySpacedConnector\",\"uuid\":\"fcafe625-79d7-4037-9431-d1cc167f79ab\"}],\"packageUris\":[\"http://schema.mathworks.com/mf0/Connector/R2020b\"],\"version\":\"1.0\"}"
  Chart_REQ_HV_ON_Batt3 : libCM/Chart_REQ_HV_ON_Batt1  SystemSampleTime=-1  VariantActivationTime=update diagram  Latency=0  AutoFrameSizeCalculation=off
      settings: PortSchema="{\"entries\":[{\"content\":{\"sides\":[{\"content\":{\"connectorIds\":[\"In1\",\"In8\",\"In2\",\"In3\",\"In4\",\"In5\",\"In6\",\"In9\",\"In10\",\"In11\",\"In15\",\"In16\",\"In12\",\"In13\",\"In14\",\"In7\",\"In17\",\"In18\"]},\"type\":\"ConnectorPlacement.EquallySpacedRectSide\",\"uuid\":\"2be98496-94d0-443a-935f-4b2e992aab8e\"},{\"content\":{\"connectorIds\":[\"Out1\",\"Out2\"],\"side\":\"RIGHT\"},\"type\":\"ConnectorPlacement.EquallySpacedRectSide\",\"uuid\":\"fda23760-2911-4bbb-ac8a-7a2dd70a4d72\"},{\"content\":{\"connectorIds\":[],\"side\":\"TOP\"},\"type\":\"ConnectorPlacement.EquallySpacedRectSide\",\"uuid\":\"77874347-bb9f-447e-8cfd-08f52997a658\"}]},\"type\":\"ConnectorPlacement.EquallySpacedConnector\",\"uuid\":\"fcafe625-79d7-4037-9431-d1cc167f79ab\"}],\"packageUris\":[\"http://schema.mathworks.com/mf0/Connector/R2020b\"],\"version\":\"1.0\"}"
  FL_u8ContactorState_BB1 : Outport
  FL_u8ContactorState_BB2 : Outport  Port=2
  FL_u8ContactorState_BB3 : Outport  Port=3
  FL_boREQ_HV_ON_BB1 : Outport  Port=4
  FL_boREQ_HV_ON_BB2 : Outport  Port=5
  FL_boREQ_HV_ON_BB3 : Outport  Port=6
  FL_u8Contactor_FB_State_BB1 : Outport  Port=7
  FL_u8Contactor_FB_State_BB2 : Outport  Port=8
  FL_u8Contactor_FB_State_BB3 : Outport  Port=9
  wires:
  IsolationMeasurementRequest/1 -> Chart_REQ_HV_ON_Batt2/17, Chart_REQ_HV_ON_Batt3/17, Chart_REQ_HV_ON_Batt1/17
  FL_boMainHV_PlusMinus_Status/1 -> Chart_REQ_HV_ON_Batt2/16, Chart_REQ_HV_ON_Batt3/13, Chart_REQ_HV_ON_Batt1/12
  HV_Plus_Sense_BB3/1 -> Chart_ContactorFB_State_Batt3/2
  HV_Minus_Sense_BB3/1 -> Chart_ContactorFB_State_Batt3/1
  HV_Plus_Sense_BB2/1 -> Chart_ContactorFB_State_Batt2/2
  HV_Minus_Sense_BB2/1 -> Chart_ContactorFB_State_Batt2/1
  FL_boSystem_SD/1 -> Chart_REQ_HV_ON_Batt2/14, Chart_REQ_HV_ON_Batt3/14, Chart_REQ_HV_ON_Batt1/14
  HV_REL_ON_BB1/1 -> Chart_REQ_HV_ON_Batt2/15, Chart_REQ_HV_ON_Batt3/15, Chart_REQ_HV_ON_Batt1/15
  SafeToSD_BB1/1 -> Chart_REQ_HV_ON_Batt2/11
  HV_REL_ON_BB3/1 -> Chart_REQ_HV_ON_Batt2/13, Chart_REQ_HV_ON_Batt3/12, Chart_REQ_HV_ON_Batt1/13
  HV_REL_ON_BB2/1 -> Chart_REQ_HV_ON_Batt2/12, Chart_REQ_HV_ON_Batt1/16, Chart_REQ_HV_ON_Batt3/16
  FL_boMainHV_SD_OK/1 -> Chart_REQ_HV_ON_Batt2/10, Chart_REQ_HV_ON_Batt1/10, Chart_REQ_HV_ON_Batt3/10
  HV_Plus_Sense_BB1/1 -> Chart_ContactorFB_State_Batt1/2
  HV_Minus_Sense_BB1/1 -> Chart_ContactorFB_State_Batt1/1
  Chart_REQ_HV_ON_Batt3/1 -> Chart_ContactorFB_State_Batt3/3, FL_boREQ_HV_ON_BB3/1
  SafeToSD_BB3/1 -> Chart_REQ_HV_ON_Batt3/11
  Chart_ContactorFB_State_Batt3/1 -> FL_u8Contactor_FB_State_BB3/1
  Chart_ContactorFB_State_Batt2/1 -> FL_u8Contactor_FB_State_BB2/1
  Chart_ContactorFB_State_Batt1/1 -> FL_u8Contactor_FB_State_BB1/1
  FL_boSafeToCloseHV_BB3/1 -> Chart_REQ_HV_ON_Batt3/9
  FL_boSafeToCloseHV_BB2/1 -> Chart_REQ_HV_ON_Batt1/9
  FL_boSafeToCloseHV_BB1/1 -> Chart_REQ_HV_ON_Batt2/9
  KL15_CM_disable/1 -> Chart_REQ_HV_ON_Batt2/8, Chart_REQ_HV_ON_Batt3/8, Chart_REQ_HV_ON_Batt1/8
  SafeToSD_BB2/1 -> Chart_REQ_HV_ON_Batt1/11
  Software_Reset_KL15_BB3/1 -> Chart_REQ_HV_ON_Batt3/7
  Software_Reset_KL15_BB2/1 -> Chart_REQ_HV_ON_Batt1/7
  Software_Reset_KL15_BB1/1 -> Chart_REQ_HV_ON_Batt2/7
  Chart_REQ_HV_ON_Batt3/2 -> FL_u8ContactorState_BB3/1  "FL_u8ContactorState_BB3"
  Chart_REQ_HV_ON_Batt1/2 -> FL_u8ContactorState_BB2/1  "FL_u8ContactorState_BB2"
  Chart_REQ_HV_ON_Batt2/2 -> FL_u8ContactorState_BB1/1  "FL_u8ContactorState_BB1"
  InsulationReadyOK_B3/1 -> Chart_REQ_HV_ON_Batt3/2
  InsulationReadyOK_B2/1 -> Chart_REQ_HV_ON_Batt1/2
  IMD_Active_BB3/1 -> Chart_REQ_HV_ON_Batt2/6, Chart_REQ_HV_ON_Batt3/6, Chart_REQ_HV_ON_Batt1/6
  IMD_Active_BB2/1 -> Chart_REQ_HV_ON_Batt2/5, Chart_REQ_HV_ON_Batt3/5, Chart_REQ_HV_ON_Batt1/5
  IMD_Active_BB1/1 -> Chart_REQ_HV_ON_Batt2/4, Chart_REQ_HV_ON_Batt3/4, Chart_REQ_HV_ON_Batt1/4
  InsulationReadyOK_B1/1 -> Chart_REQ_HV_ON_Batt2/2
  Chart_REQ_HV_ON_Batt1/1 -> Chart_ContactorFB_State_Batt2/3, FL_boREQ_HV_ON_BB2/1
  Chart_REQ_HV_ON_Batt2/1 -> Chart_ContactorFB_State_Batt1/3, FL_boREQ_HV_ON_BB1/1
  SDError_BB3/1 -> Chart_REQ_HV_ON_Batt3/3
  SDError_BB2/1 -> Chart_REQ_HV_ON_Batt1/3
  SDError_BB1/1 -> Chart_REQ_HV_ON_Batt2/3
  FL_boST_REQ_HV_Open_BB1/1 -> Chart_REQ_HV_ON_Batt2/18
  FL_boST_REQ_HV_Open_BB2/1 -> Chart_REQ_HV_ON_Batt1/18
  FL_boST_REQ_HV_Open_BB3/1 -> Chart_REQ_HV_ON_Batt3/18
  IP_boChargeStop_Pressed/1 -> Chart_REQ_HV_ON_Batt2/1, Chart_REQ_HV_ON_Batt3/1, Chart_REQ_HV_ON_Batt1/1
